simulink model "final_quadruped_040622"  (R2021a)
settings: Solver=FixedStepAuto  StartTime=0.0  StopTime=5  FixedStep=.001  RelTol=1e-3  EnableMultiTasking=on
values from neighbouring files (symbols this model uses):
  foot_x = 8    [bipedparameters.m]    (also in fcn.m; finalrobotParameters.m; finalrobotParameters_110522.m; finalrobotParameters_140522.m)
  foot_y = 6    [bipedparameters.m]    (also in fcn.m; finalrobotParameters.m; finalrobotParameters_110522.m; finalrobotParameters_140522.m)
  foot_z = 1    [bipedparameters.m]    (also in fcn.m; finalrobotParameters.m; finalrobotParameters_110522.m; finalrobotParameters_140522.m)
  height_plane = 0.025    [bipedparameters.m]    (also in finalrobotParameters.m; finalrobotParameters_110522.m; finalrobotParameters_140522.m; finalrobotParameters_240522.m)
  kd_ankle = 1000    [bipedparameters.m]    (also in finalrobotParameters_240522.m)
  kd_hip = 1000    [bipedparameters.m]    (also in finalrobotParameters_240522.m)
  kd_knee = 1000    [bipedparameters.m]    (also in finalrobotParameters_240522.m)
  ki_ankle = 1000    [bipedparameters.m]    (also in finalrobotParameters_240522.m)
  ki_hip = 1000    [bipedparameters.m]    (also in finalrobotParameters_240522.m)
  ki_knee = 2000    [bipedparameters.m]    (also in finalrobotParameters_240522.m)
  kp_ankle = 1000    [bipedparameters.m]    (also in finalrobotParameters_240522.m)
  kp_hip = 1000    [bipedparameters.m]    (also in finalrobotParameters_240522.m)
  kp_knee = 2000    [bipedparameters.m]    (also in finalrobotParameters_240522.m)
  lower_leg_length = 10    [bipedparameters.m]    (also in fcn.m; finalrobotParameters.m; finalrobotParameters_110522.m; finalrobotParameters_140522.m)
  m_ll = density*leg_radius*leg_radius*lower_leg_length*3.141592653589*0.01*0.01*0.01    (= 0.0176714586764)    [bipedparameters.m]    (also in fcn.m; finalrobotParameters_140522.m; finalrobotParameters_240522.m; hdotlb.m)
  m_ul = density*leg_radius*leg_radius*upper_leg_length*3.141592653589*0.01*0.01*0.01    (= 0.0176714586764)    [bipedparameters.m]    (also in fcn.m; finalrobotParameters_140522.m; finalrobotParameters_240522.m; hdotlb.m)
  plane_x = 25    [bipedparameters.m]    (also in finalrobotParameters.m; finalrobotParameters_110522.m; finalrobotParameters_140522.m; finalrobotParameters_240522.m)
  plane_y = 3    [bipedparameters.m]    (also in finalrobotParameters.m; finalrobotParameters_110522.m; finalrobotParameters_140522.m; finalrobotParameters_240522.m)
  torso_offset_x = -0.5    [bipedparameters.m]    (also in finalrobotParameters.m = 10; finalrobotParameters_110522.m = 10; finalrobotParameters_140522.m = 10; finalrobotParameters_240522.m = 10)
  torso_offset_z = -2    [bipedparameters.m]    (also in finalrobotParameters.m; finalrobotParameters_110522.m; finalrobotParameters_140522.m; finalrobotParameters_240522.m)
  torso_x = 5    [bipedparameters.m]    (also in fcn.m = 25; finalrobotParameters.m = 25; finalrobotParameters_110522.m = 25; finalrobotParameters_140522.m = 25)
  torso_y = 10    [bipedparameters.m]    (also in fcn.m = 16; finalrobotParameters.m = 16; finalrobotParameters_110522.m = 16; finalrobotParameters_140522.m = 16)
  torso_z = 8    [bipedparameters.m]    (also in fcn.m = 10; finalrobotParameters.m = 10; finalrobotParameters_110522.m = 10; finalrobotParameters_140522.m = 10)
  upper_leg_length = 10    [bipedparameters.m]    (also in fcn.m; finalrobotParameters.m; finalrobotParameters_110522.m; finalrobotParameters_140522.m)
undefined symbols (not defined in the file or in its folder): angleLFhip, speedLFhip, torqueLFhip, X, Y, Z
libraries: nesl_utility x151, sm_lib x71, Contact_Forces_Lib x16, pid_lib x12, fl_lib x4
(part 2 of 7)

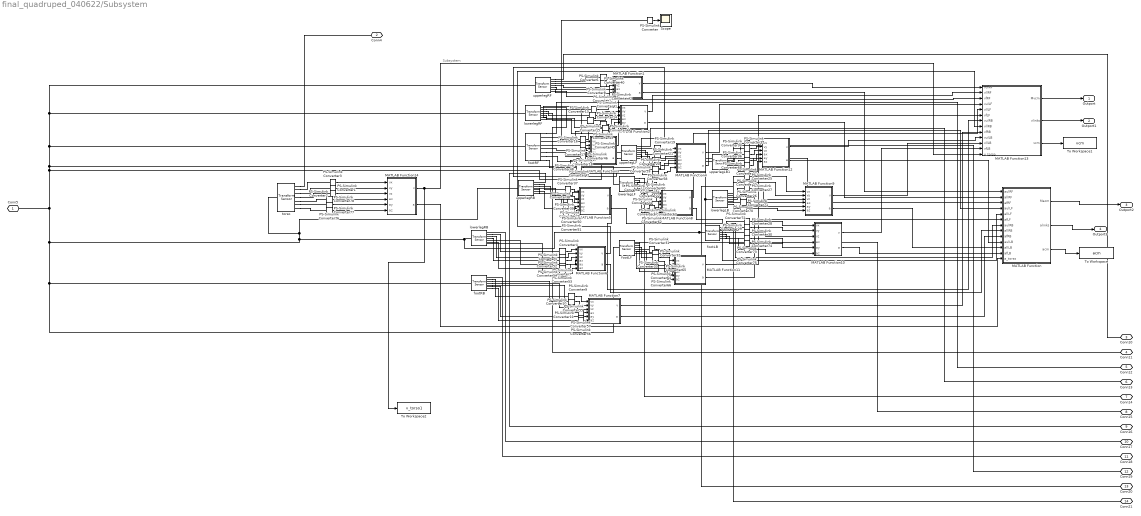
== system final_quadruped_040622/Subsystem ==
  note: Subsystem
  MATLAB Function : MATLAB Function  TreatAsAtomicUnit=on
  MATLAB Function1 : MATLAB Function  TreatAsAtomicUnit=on
  MATLAB Function10 : MATLAB Function  TreatAsAtomicUnit=on
  MATLAB Function11 : MATLAB Function  TreatAsAtomicUnit=on
  MATLAB Function12 : MATLAB Function  TreatAsAtomicUnit=on
  MATLAB Function13 : MATLAB Function  TreatAsAtomicUnit=on
  MATLAB Function14 : MATLAB Function  TreatAsAtomicUnit=on
  MATLAB Function2 : MATLAB Function  TreatAsAtomicUnit=on
  MATLAB Function3 : MATLAB Function  TreatAsAtomicUnit=on
  MATLAB Function4 : MATLAB Function  TreatAsAtomicUnit=on
  MATLAB Function5 : MATLAB Function  TreatAsAtomicUnit=on
  MATLAB Function6 : MATLAB Function  TreatAsAtomicUnit=on
  MATLAB Function7 : MATLAB Function  TreatAsAtomicUnit=on
  MATLAB Function8 : MATLAB Function  TreatAsAtomicUnit=on
  MATLAB Function9 : MATLAB Function  TreatAsAtomicUnit=on
  PS-Simulink Converter{,1..78} (79 alike) : nesl_utility/PS-Simulink Converter  PhysicalDomain=network_engine_domain  SubClassName=ps_output  LeftPortType=input  RightPortType=output  PseudoPeriodic=off  Frequencies=[]  Unit=inherit  AffineConversion=off
      settings: SourceProductBaseCode=PW,SS
  Scope : Scope
  To Workspace : ToWorkspace  VariableName=acm  SaveFormat=Timeseries  SampleTime=-1
  To Workspace1 : ToWorkspace  VariableName=vcm  SaveFormat=Timeseries  SampleTime=-1
  To Workspace2 : ToWorkspace  VariableName=v_torso1  SaveFormat=Timeseries  SampleTime=-1
  footLB : sm_lib/Frames and Transforms/Transform Sensor  MeasurementFrame=World  SenseAngle=off  SenseAxis=off  SenseAngle1=off  SenseAngle2=off  SenseAngle3=off  SenseQ=off  SenseR=off  SenseOmegaX=off  SenseOmegaY=off  SenseOmegaZ=off  SenseOmega1=off  SenseOmega2=off  SenseOmega3=off  SenseQDot=off  SenseRDot=off  SenseAlphaX=off  SenseAlphaY=off  SenseAlphaZ=off  SenseAlpha1=off  SenseAlpha2=off  SenseAlpha3=off  SenseQDDot=off  SenseRDDot=off  SenseX=off  SenseY=off  SenseZ=off  SenseRad=off  SenseAzim=off  SenseDist=off  SenseInc=off  SenseXDot=on  SenseYDot=on  SenseZDot=on  SenseRadDot=off  SenseAzimDot=off  SenseDistDot=off  SenseIncDot=off  SenseXDDot=on  SenseYDDot=on  SenseZDDot=on  SenseRadDDot=off  SenseAzimDDot=off  SenseDistDDot=off  SenseIncDDot=off
  footLF : sm_lib/Frames and Transforms/Transform Sensor  MeasurementFrame=World  SenseAngle=off  SenseAxis=off  SenseAngle1=off  SenseAngle2=off  SenseAngle3=off  SenseQ=off  SenseR=off  SenseOmegaX=off  SenseOmegaY=off  SenseOmegaZ=off  SenseOmega1=off  SenseOmega2=off  SenseOmega3=off  SenseQDot=off  SenseRDot=off  SenseAlphaX=off  SenseAlphaY=off  SenseAlphaZ=off  SenseAlpha1=off  SenseAlpha2=off  SenseAlpha3=off  SenseQDDot=off  SenseRDDot=off  SenseX=off  SenseY=off  SenseZ=off  SenseRad=off  SenseAzim=off  SenseDist=off  SenseInc=off  SenseXDot=on  SenseYDot=on  SenseZDot=on  SenseRadDot=off  SenseAzimDot=off  SenseDistDot=off  SenseIncDot=off  SenseXDDot=on  SenseYDDot=on  SenseZDDot=on  SenseRadDDot=off  SenseAzimDDot=off  SenseDistDDot=off  SenseIncDDot=off
  footRB : sm_lib/Frames and Transforms/Transform Sensor  MeasurementFrame=World  SenseAngle=off  SenseAxis=off  SenseAngle1=off  SenseAngle2=off  SenseAngle3=off  SenseQ=off  SenseR=off  SenseOmegaX=off  SenseOmegaY=off  SenseOmegaZ=off  SenseOmega1=off  SenseOmega2=off  SenseOmega3=off  SenseQDot=off  SenseRDot=off  SenseAlphaX=off  SenseAlphaY=off  SenseAlphaZ=off  SenseAlpha1=off  SenseAlpha2=off  SenseAlpha3=off  SenseQDDot=off  SenseRDDot=off  SenseX=off  SenseY=off  SenseZ=off  SenseRad=off  SenseAzim=off  SenseDist=off  SenseInc=off  SenseXDot=on  SenseYDot=on  SenseZDot=on  SenseRadDot=off  SenseAzimDot=off  SenseDistDot=off  SenseIncDot=off  SenseXDDot=on  SenseYDDot=on  SenseZDDot=on  SenseRadDDot=off  SenseAzimDDot=off  SenseDistDDot=off  SenseIncDDot=off
  footRF : sm_lib/Frames and Transforms/Transform Sensor  MeasurementFrame=World  SenseAngle=on  SenseAxis=off  SenseAngle1=off  SenseAngle2=off  SenseAngle3=off  SenseQ=off  SenseR=off  SenseOmegaX=off  SenseOmegaY=off  SenseOmegaZ=off  SenseOmega1=off  SenseOmega2=off  SenseOmega3=off  SenseQDot=off  SenseRDot=off  SenseAlphaX=off  SenseAlphaY=off  SenseAlphaZ=off  SenseAlpha1=off  SenseAlpha2=off  SenseAlpha3=off  SenseQDDot=off  SenseRDDot=off  SenseX=off  SenseY=off  SenseZ=off  SenseRad=off  SenseAzim=off  SenseDist=off  SenseInc=off  SenseXDot=on  SenseYDot=on  SenseZDot=on  SenseRadDot=off  SenseAzimDot=off  SenseDistDot=off  SenseIncDot=off  SenseXDDot=on  SenseYDDot=on  SenseZDDot=on  SenseRadDDot=off  SenseAzimDDot=off  SenseDistDDot=off  SenseIncDDot=off
  lowerlegLB : sm_lib/Frames and Transforms/Transform Sensor  MeasurementFrame=World  SenseAngle=off  SenseAxis=off  SenseAngle1=off  SenseAngle2=off  SenseAngle3=off  SenseQ=off  SenseR=off  SenseOmegaX=off  SenseOmegaY=off  SenseOmegaZ=off  SenseOmega1=off  SenseOmega2=off  SenseOmega3=off  SenseQDot=off  SenseRDot=off  SenseAlphaX=off  SenseAlphaY=off  SenseAlphaZ=off  SenseAlpha1=off  SenseAlpha2=off  SenseAlpha3=off  SenseQDDot=off  SenseRDDot=off  SenseX=off  SenseY=off  SenseZ=off  SenseRad=off  SenseAzim=off  SenseDist=off  SenseInc=off  SenseXDot=on  SenseYDot=on  SenseZDot=on  SenseRadDot=off  SenseAzimDot=off  SenseDistDot=off  SenseIncDot=off  SenseXDDot=on  SenseYDDot=on  SenseZDDot=on  SenseRadDDot=off  SenseAzimDDot=off  SenseDistDDot=off  SenseIncDDot=off
  lowerlegLF : sm_lib/Frames and Transforms/Transform Sensor  MeasurementFrame=World  SenseAngle=off  SenseAxis=off  SenseAngle1=off  SenseAngle2=off  SenseAngle3=off  SenseQ=off  SenseR=off  SenseOmegaX=off  SenseOmegaY=off  SenseOmegaZ=off  SenseOmega1=off  SenseOmega2=off  SenseOmega3=off  SenseQDot=off  SenseRDot=off  SenseAlphaX=off  SenseAlphaY=off  SenseAlphaZ=off  SenseAlpha1=off  SenseAlpha2=off  SenseAlpha3=off  SenseQDDot=off  SenseRDDot=off  SenseX=off  SenseY=off  SenseZ=off  SenseRad=off  SenseAzim=off  SenseDist=off  SenseInc=off  SenseXDot=on  SenseYDot=on  SenseZDot=on  SenseRadDot=off  SenseAzimDot=off  SenseDistDot=off  SenseIncDot=off  SenseXDDot=on  SenseYDDot=on  SenseZDDot=on  SenseRadDDot=off  SenseAzimDDot=off  SenseDistDDot=off  SenseIncDDot=off
  lowerlegRB : sm_lib/Frames and Transforms/Transform Sensor  MeasurementFrame=World  SenseAngle=off  SenseAxis=off  SenseAngle1=off  SenseAngle2=off  SenseAngle3=off  SenseQ=off  SenseR=off  SenseOmegaX=off  SenseOmegaY=off  SenseOmegaZ=off  SenseOmega1=off  SenseOmega2=off  SenseOmega3=off  SenseQDot=off  SenseRDot=off  SenseAlphaX=off  SenseAlphaY=off  SenseAlphaZ=off  SenseAlpha1=off  SenseAlpha2=off  SenseAlpha3=off  SenseQDDot=off  SenseRDDot=off  SenseX=off  SenseY=off  SenseZ=off  SenseRad=off  SenseAzim=off  SenseDist=off  SenseInc=off  SenseXDot=on  SenseYDot=on  SenseZDot=on  SenseRadDot=off  SenseAzimDot=off  SenseDistDot=off  SenseIncDot=off  SenseXDDot=on  SenseYDDot=on  SenseZDDot=on  SenseRadDDot=off  SenseAzimDDot=off  SenseDistDDot=off  SenseIncDDot=off
  lowerlegRF : sm_lib/Frames and Transforms/Transform Sensor  MeasurementFrame=World  SenseAngle=off  SenseAxis=off  SenseAngle1=off  SenseAngle2=off  SenseAngle3=off  SenseQ=off  SenseR=off  SenseOmegaX=off  SenseOmegaY=off  SenseOmegaZ=off  SenseOmega1=off  SenseOmega2=off  SenseOmega3=off  SenseQDot=off  SenseRDot=off  SenseAlphaX=off  SenseAlphaY=off  SenseAlphaZ=off  SenseAlpha1=off  SenseAlpha2=off  SenseAlpha3=off  SenseQDDot=off  SenseRDDot=off  SenseX=off  SenseY=off  SenseZ=off  SenseRad=off  SenseAzim=off  SenseDist=off  SenseInc=off  SenseXDot=on  SenseYDot=on  SenseZDot=on  SenseRadDot=off  SenseAzimDot=off  SenseDistDot=off  SenseIncDot=off  SenseXDDot=on  SenseYDDot=on  SenseZDDot=on  SenseRadDDot=off  SenseAzimDDot=off  SenseDistDDot=off  SenseIncDDot=off
  torso : sm_lib/Frames and Transforms/Transform Sensor  MeasurementFrame=World  SenseAngle=off  SenseAxis=off  SenseAngle1=off  SenseAngle2=off  SenseAngle3=off  SenseQ=off  SenseR=off  SenseOmegaX=off  SenseOmegaY=off  SenseOmegaZ=off  SenseOmega1=off  SenseOmega2=off  SenseOmega3=off  SenseQDot=off  SenseRDot=off  SenseAlphaX=off  SenseAlphaY=off  SenseAlphaZ=off  SenseAlpha1=off  SenseAlpha2=off  SenseAlpha3=off  SenseQDDot=off  SenseRDDot=off  SenseX=off  SenseY=off  SenseZ=off  SenseRad=off  SenseAzim=off  SenseDist=off  SenseInc=off  SenseXDot=on  SenseYDot=on  SenseZDot=on  SenseRadDot=off  SenseAzimDot=off  SenseDistDot=off  SenseIncDot=off  SenseXDDot=on  SenseYDDot=on  SenseZDDot=on  SenseRadDDot=off  SenseAzimDDot=off  SenseDistDDot=off  SenseIncDDot=off
  upperlegLB1 : sm_lib/Frames and Transforms/Transform Sensor  MeasurementFrame=World  SenseAngle=off  SenseAxis=off  SenseAngle1=off  SenseAngle2=off  SenseAngle3=off  SenseQ=off  SenseR=off  SenseOmegaX=off  SenseOmegaY=off  SenseOmegaZ=off  SenseOmega1=off  SenseOmega2=off  SenseOmega3=off  SenseQDot=off  SenseRDot=off  SenseAlphaX=off  SenseAlphaY=off  SenseAlphaZ=off  SenseAlpha1=off  SenseAlpha2=off  SenseAlpha3=off  SenseQDDot=off  SenseRDDot=off  SenseX=off  SenseY=off  SenseZ=off  SenseRad=off  SenseAzim=off  SenseDist=off  SenseInc=off  SenseXDot=on  SenseYDot=on  SenseZDot=on  SenseRadDot=off  SenseAzimDot=off  SenseDistDot=off  SenseIncDot=off  SenseXDDot=on  SenseYDDot=on  SenseZDDot=on  SenseRadDDot=off  SenseAzimDDot=off  SenseDistDDot=off  SenseIncDDot=off
  upperlegLF : sm_lib/Frames and Transforms/Transform Sensor  MeasurementFrame=World  SenseAngle=off  SenseAxis=off  SenseAngle1=off  SenseAngle2=off  SenseAngle3=off  SenseQ=off  SenseR=off  SenseOmegaX=off  SenseOmegaY=off  SenseOmegaZ=off  SenseOmega1=off  SenseOmega2=off  SenseOmega3=off  SenseQDot=off  SenseRDot=off  SenseAlphaX=off  SenseAlphaY=off  SenseAlphaZ=off  SenseAlpha1=off  SenseAlpha2=off  SenseAlpha3=off  SenseQDDot=off  SenseRDDot=off  SenseX=off  SenseY=off  SenseZ=off  SenseRad=off  SenseAzim=off  SenseDist=off  SenseInc=off  SenseXDot=on  SenseYDot=on  SenseZDot=on  SenseRadDot=off  SenseAzimDot=off  SenseDistDot=off  SenseIncDot=off  SenseXDDot=on  SenseYDDot=on  SenseZDDot=on  SenseRadDDot=off  SenseAzimDDot=off  SenseDistDDot=off  SenseIncDDot=off
  upperlegRB : sm_lib/Frames and Transforms/Transform Sensor  MeasurementFrame=World  SenseAngle=off  SenseAxis=off  SenseAngle1=off  SenseAngle2=off  SenseAngle3=off  SenseQ=off  SenseR=off  SenseOmegaX=off  SenseOmegaY=off  SenseOmegaZ=off  SenseOmega1=off  SenseOmega2=off  SenseOmega3=off  SenseQDot=off  SenseRDot=off  SenseAlphaX=off  SenseAlphaY=off  SenseAlphaZ=off  SenseAlpha1=off  SenseAlpha2=off  SenseAlpha3=off  SenseQDDot=off  SenseRDDot=off  SenseX=off  SenseY=off  SenseZ=off  SenseRad=off  SenseAzim=off  SenseDist=off  SenseInc=off  SenseXDot=on  SenseYDot=on  SenseZDot=on  SenseRadDot=off  SenseAzimDot=off  SenseDistDot=off  SenseIncDot=off  SenseXDDot=on  SenseYDDot=on  SenseZDDot=on  SenseRadDDot=off  SenseAzimDDot=off  SenseDistDDot=off  SenseIncDDot=off
  upperlegRF : sm_lib/Frames and Transforms/Transform Sensor  MeasurementFrame=World  SenseAngle=off  SenseAxis=off  SenseAngle1=off  SenseAngle2=off  SenseAngle3=off  SenseQ=off  SenseR=off  SenseOmegaX=off  SenseOmegaY=off  SenseOmegaZ=off  SenseOmega1=off  SenseOmega2=off  SenseOmega3=off  SenseQDot=off  SenseRDot=off  SenseAlphaX=off  SenseAlphaY=off  SenseAlphaZ=off  SenseAlpha1=off  SenseAlpha2=off  SenseAlpha3=off  SenseQDDot=off  SenseRDDot=off  SenseX=off  SenseY=off  SenseZ=off  SenseRad=off  SenseAzim=off  SenseDist=off  SenseInc=off  SenseXDot=on  SenseYDot=on  SenseZDot=on  SenseRadDot=off  SenseAzimDot=off  SenseDistDot=off  SenseIncDot=off  SenseXDDot=on  SenseYDDot=on  SenseZDDot=on  SenseRadDDot=off  SenseAzimDDot=off  SenseDistDDot=off  SenseIncDDot=off
  Conn5 : PMIOPort  Side=Left
  Conn4 : PMIOPort  Port=2  Side=Right
  Conn10 : PMIOPort  Port=3  Side=Right
  Conn11 : PMIOPort  Port=4  Side=Right
  Conn12 : PMIOPort  Port=5  Side=Right
  Conn13 : PMIOPort  Port=6  Side=Right
  Conn14 : PMIOPort  Port=7  Side=Right
  Conn15 : PMIOPort  Port=8  Side=Right
  Conn16 : PMIOPort  Port=9  Side=Right
  Conn17 : PMIOPort  Port=10  Side=Right
  Conn18 : PMIOPort  Port=11  Side=Right
  Conn19 : PMIOPort  Port=12  Side=Right
  Conn20 : PMIOPort  Port=13  Side=Right
  Conn21 : PMIOPort  Port=14  Side=Right
  Outport : Outport
  Outport1 : Outport  Port=2
  Outport2 : Outport  Port=3
  Outport3 : Outport  Port=4
  wires:
  PS-Simulink Converter10/1 -> MATLAB Function7/2(vy)
  PS-Simulink Converter13/1 -> MATLAB Function2/1(vx)
  MATLAB Function12/1(v) -> MATLAB Function13/10(vulLB)
  PS-Simulink Converter36/1 -> MATLAB Function12/3(vz)
  PS-Simulink Converter14/1 -> MATLAB Function2/2(vy)
  PS-Simulink Converter9/1 -> MATLAB Function7/1(vx)
  PS-Simulink Converter11/1 -> MATLAB Function7/3(vz)
  PS-Simulink Converter8/1 -> MATLAB Function1/2(vy)
  PS-Simulink Converter7/1 -> MATLAB Function6/3(vz)
  PS-Simulink Converter38/1 -> MATLAB Function5/2(vy)
  PS-Simulink Converter16/1 -> MATLAB Function3/1(vx)
  MATLAB Function9/1(v) -> MATLAB Function13/11(vllLB)
  MATLAB Function1/1(v) -> MATLAB Function13/1(vulRF)
  PS-Simulink Converter17/1 -> MATLAB Function3/2(vy)
  PS-Simulink Converter28/1 -> MATLAB Function10/1(vx)
  PS-Simulink Converter21/1 -> MATLAB Function4/3(vz)
  PS-Simulink Converter18/1 -> MATLAB Function3/3(vz)
  PS-Simulink Converter6/1 -> MATLAB Function1/1(vx)
  PS-Simulink Converter19/1 -> MATLAB Function4/1(vx)
  PS-Simulink Converter5/1 -> MATLAB Function6/2(vy)
  PS-Simulink Converter20/1 -> MATLAB Function4/2(vy)
  PS-Simulink Converter12/1 -> MATLAB Function1/3(vz)
  PS-Simulink Converter15/1 -> MATLAB Function2/3(vz)
  PS-Simulink Converter39/1 -> MATLAB Function5/3(vz)
  MATLAB Function2/1(v) -> MATLAB Function13/2(vllRF)
  MATLAB Function10/1(v) -> MATLAB Function13/12(vfLB)
  PS-Simulink Converter27/1 -> MATLAB Function9/3(vz)
  PS-Simulink Converter4/1 -> MATLAB Function6/1(vx)
  PS-Simulink Converter25/1 -> MATLAB Function9/1(vx)
  PS-Simulink Converter37/1 -> MATLAB Function5/1(vx)
  PS-Simulink Converter26/1 -> MATLAB Function9/2(vy)
  PS-Simulink Converter24/1 -> MATLAB Function8/3(vz)
  PS-Simulink Converter22/1 -> MATLAB Function8/1(vx)
  PS-Simulink Converter23/1 -> MATLAB Function8/2(vy)
  PS-Simulink Converter34/1 -> MATLAB Function12/1(vx)
  PS-Simulink Converter35/1 -> MATLAB Function12/2(vy)
  MATLAB Function7/1(v) -> MATLAB Function13/9(vfRB)
  MATLAB Function6/1(v) -> MATLAB Function13/8(vllRB)
  MATLAB Function5/1(v) -> MATLAB Function13/7(vulRB)
  MATLAB Function11/1(v) -> MATLAB Function13/6(vfLF)
  PS-Simulink Converter33/1 -> MATLAB Function11/3(vz)
  MATLAB Function8/1(v) -> MATLAB Function13/5(vllLF)
  MATLAB Function4/1(v) -> MATLAB Function13/4(vulLF)
  MATLAB Function3/1(v) -> MATLAB Function13/3(vfRF)
  PS-Simulink Converter32/1 -> MATLAB Function11/2(vy)
  PS-Simulink Converter31/1 -> MATLAB Function11/1(vx)
  PS-Simulink Converter30/1 -> MATLAB Function10/3(vz)
  PS-Simulink Converter29/1 -> MATLAB Function10/2(vy)
  PS-Simulink Converter3/1 -> MATLAB Function14/1(vx)
  PS-Simulink Converter1/1 -> MATLAB Function14/2(vy)
  PS-Simulink Converter2/1 -> MATLAB Function14/3(vz)
  MATLAB Function14/1(v) -> To Workspace2/1, MATLAB Function13/13(v_torso)
  MATLAB Function13/1(Mvcm) -> Outport/1
  MATLAB Function13/2(vlinks) -> Outport1/1
  PS-Simulink Converter/1 -> Scope/1
  PS-Simulink Converter40/1 -> MATLAB Function1/4(ax)
  PS-Simulink Converter41/1 -> MATLAB Function1/5(ay)
  PS-Simulink Converter42/1 -> MATLAB Function1/6(az)
  PS-Simulink Converter43/1 -> MATLAB Function2/4(ax)
  PS-Simulink Converter44/1 -> MATLAB Function2/5(ay)
  PS-Simulink Converter45/1 -> MATLAB Function2/6(az)
  PS-Simulink Converter46/1 -> MATLAB Function3/4(ax)
  PS-Simulink Converter47/1 -> MATLAB Function3/5(ay)
  PS-Simulink Converter48/1 -> MATLAB Function3/6(az)
  PS-Simulink Converter49/1 -> MATLAB Function5/4(ax)
  PS-Simulink Converter50/1 -> MATLAB Function5/5(ay)
  PS-Simulink Converter51/1 -> MATLAB Function5/6(az)
  PS-Simulink Converter52/1 -> MATLAB Function6/4(ax)
  PS-Simulink Converter53/1 -> MATLAB Function6/5(ay)
  PS-Simulink Converter54/1 -> MATLAB Function6/6(az)
  PS-Simulink Converter55/1 -> MATLAB Function7/5(ay)
  PS-Simulink Converter57/1 -> MATLAB Function7/4(ax)
  PS-Simulink Converter56/1 -> MATLAB Function7/6(az)
  PS-Simulink Converter58/1 -> MATLAB Function4/4(ax)
  PS-Simulink Converter59/1 -> MATLAB Function4/5(ay)
  PS-Simulink Converter60/1 -> MATLAB Function4/6(az)
  PS-Simulink Converter61/1 -> MATLAB Function8/4(ax)
  PS-Simulink Converter62/1 -> MATLAB Function8/5(ay)
  PS-Simulink Converter63/1 -> MATLAB Function8/6(az)
  PS-Simulink Converter64/1 -> MATLAB Function11/4(ax)
  PS-Simulink Converter65/1 -> MATLAB Function11/5(ay)
  PS-Simulink Converter66/1 -> MATLAB Function11/6(az)
  PS-Simulink Converter67/1 -> MATLAB Function12/4(ax)
  PS-Simulink Converter68/1 -> MATLAB Function12/5(ay)
  PS-Simulink Converter69/1 -> MATLAB Function12/6(az)
  PS-Simulink Converter70/1 -> MATLAB Function9/4(ax)
  PS-Simulink Converter71/1 -> MATLAB Function9/5(ay)
  PS-Simulink Converter72/1 -> MATLAB Function9/6(az)
  PS-Simulink Converter73/1 -> MATLAB Function10/4(ax)
  PS-Simulink Converter74/1 -> MATLAB Function10/5(ay)
  PS-Simulink Converter75/1 -> MATLAB Function10/6(az)
  PS-Simulink Converter78/1 -> MATLAB Function14/4(ax)
  PS-Simulink Converter76/1 -> MATLAB Function14/5(ay)
  PS-Simulink Converter77/1 -> MATLAB Function14/6(az)
  MATLAB Function14/2(a) -> MATLAB Function/13(a_torso)
  MATLAB Function1/2(a) -> MATLAB Function/1(aulRF)
  MATLAB Function2/2(a) -> MATLAB Function/2(allRF)
  MATLAB Function3/2(a) -> MATLAB Function/3(afRF)
  MATLAB Function4/2(a) -> MATLAB Function/4(aulLF)
  MATLAB Function8/2(a) -> MATLAB Function/5(allLF)
  MATLAB Function11/2(a) -> MATLAB Function/6(afLF)
  MATLAB Function5/2(a) -> MATLAB Function/7(aulRB)
  MATLAB Function6/2(a) -> MATLAB Function/8(allRB)
  MATLAB Function7/2(a) -> MATLAB Function/9(afRB)
  MATLAB Function12/2(a) -> MATLAB Function/10(aulLB)
  MATLAB Function9/2(a) -> MATLAB Function/11(allLB)
  MATLAB Function10/2(a) -> MATLAB Function/12(afLB)
  MATLAB Function/1(Macm) -> Outport2/1
  MATLAB Function/2(alinks) -> Outport3/1
  MATLAB Function/3(acm) -> To Workspace/1
  MATLAB Function13/3(vcm) -> To Workspace1/1
  connections:
  footRB/RConn4 -- PS-Simulink Converter11/LConn1
  lowerlegLF/RConn2 -- PS-Simulink Converter22/LConn1
  upperlegLF/RConn4 -- PS-Simulink Converter21/LConn1
  footLB/RConn2 -- PS-Simulink Converter28/LConn1
  upperlegLB1/RConn1 -- Conn19/RConn1
  footLF/RConn2 -- PS-Simulink Converter31/LConn1
  lowerlegLB/LConn1 -- upperlegLB1/LConn1 -- footLB/LConn1 -- torso/LConn1 -- upperlegRB/LConn1 -- footLF/LConn1 -- footRB/LConn1 -- upperlegRF/LConn1 -- lowerlegRF/LConn1 -- footRF/LConn1 -- lowerlegLF/LConn1 -- upperlegLF/LConn1 -- Conn5/RConn1 -- lowerlegRB/LConn1
  lowerlegRB/RConn4 -- PS-Simulink Converter7/LConn1
  Conn17/RConn1 -- lowerlegRB/RConn1
  upperlegLF/RConn2 -- PS-Simulink Converter19/LConn1
  upperlegLF/RConn3 -- PS-Simulink Converter20/LConn1
  lowerlegRF/RConn3 -- PS-Simulink Converter14/LConn1
  footLB/RConn4 -- PS-Simulink Converter30/LConn1
  footRB/RConn3 -- PS-Simulink Converter10/LConn1
  upperlegRB/RConn3 -- PS-Simulink Converter38/LConn1
  lowerlegRF/RConn2 -- PS-Simulink Converter13/LConn1
  upperlegRB/RConn4 -- PS-Simulink Converter39/LConn1
  upperlegRB/RConn2 -- PS-Simulink Converter37/LConn1
  upperlegRF/RConn2 -- PS-Simulink Converter6/LConn1
  footLB/RConn1 -- Conn21/RConn1
  lowerlegRF/RConn4 -- PS-Simulink Converter15/LConn1
  lowerlegLF/RConn4 -- PS-Simulink Converter24/LConn1
  upperlegLB1/RConn4 -- PS-Simulink Converter36/LConn1
  footRB/RConn2 -- PS-Simulink Converter9/LConn1
  upperlegRF/RConn4 -- PS-Simulink Converter12/LConn1
  upperlegRF/RConn3 -- PS-Simulink Converter8/LConn1
  lowerlegLF/RConn3 -- PS-Simulink Converter23/LConn1
  lowerlegRB/RConn3 -- PS-Simulink Converter5/LConn1
  lowerlegRB/RConn2 -- PS-Simulink Converter4/LConn1
  lowerlegLB/RConn3 -- PS-Simulink Converter26/LConn1
  lowerlegLB/RConn4 -- PS-Simulink Converter27/LConn1
  lowerlegLB/RConn2 -- PS-Simulink Converter25/LConn1
  lowerlegLB/RConn1 -- Conn20/RConn1
  upperlegLB1/RConn3 -- PS-Simulink Converter35/LConn1
  upperlegLB1/RConn2 -- PS-Simulink Converter34/LConn1
  upperlegRF/RConn1 -- Conn10/RConn1
  upperlegLF/RConn1 -- Conn13/RConn1
  footLF/RConn3 -- PS-Simulink Converter32/LConn1
  footLF/RConn4 -- PS-Simulink Converter33/LConn1
  footLB/RConn3 -- PS-Simulink Converter29/LConn1
  Conn18/RConn1 -- footRB/RConn1
  footLF/RConn1 -- Conn15/RConn1
  Conn16/RConn1 -- upperlegRB/RConn1
  lowerlegLF/RConn1 -- Conn14/RConn1
  Conn11/RConn1 -- lowerlegRF/RConn1
  footRF/RConn1 -- Conn12/RConn1
  torso/RConn1 -- Conn4/RConn1
  torso/RConn3 -- PS-Simulink Converter1/LConn1
  torso/RConn2 -- PS-Simulink Converter3/LConn1
  torso/RConn4 -- PS-Simulink Converter2/LConn1
  PS-Simulink Converter16/LConn1 -- footRF/RConn3
  PS-Simulink Converter17/LConn1 -- footRF/RConn4
  PS-Simulink Converter18/LConn1 -- footRF/RConn5
  PS-Simulink Converter/LConn1 -- footRF/RConn2
  upperlegRF/RConn5 -- PS-Simulink Converter40/LConn1
  upperlegRF/RConn6 -- PS-Simulink Converter41/LConn1
  upperlegRF/RConn7 -- PS-Simulink Converter42/LConn1
  lowerlegRF/RConn5 -- PS-Simulink Converter43/LConn1
  lowerlegRF/RConn6 -- PS-Simulink Converter44/LConn1
  lowerlegRF/RConn7 -- PS-Simulink Converter45/LConn1
  footRF/RConn6 -- PS-Simulink Converter46/LConn1
  footRF/RConn7 -- PS-Simulink Converter47/LConn1
  footRF/RConn8 -- PS-Simulink Converter48/LConn1
  upperlegRB/RConn5 -- PS-Simulink Converter49/LConn1
  upperlegRB/RConn6 -- PS-Simulink Converter50/LConn1
  upperlegRB/RConn7 -- PS-Simulink Converter51/LConn1
  PS-Simulink Converter52/LConn1 -- lowerlegRB/RConn5
  PS-Simulink Converter53/LConn1 -- lowerlegRB/RConn6
  PS-Simulink Converter54/LConn1 -- lowerlegRB/RConn7
  footRB/RConn5 -- PS-Simulink Converter57/LConn1
  footRB/RConn6 -- PS-Simulink Converter55/LConn1
  footRB/RConn7 -- PS-Simulink Converter56/LConn1
  upperlegLF/RConn5 -- PS-Simulink Converter58/LConn1
  upperlegLF/RConn6 -- PS-Simulink Converter59/LConn1
  upperlegLF/RConn7 -- PS-Simulink Converter60/LConn1
  lowerlegLF/RConn5 -- PS-Simulink Converter61/LConn1
  lowerlegLF/RConn6 -- PS-Simulink Converter62/LConn1
  lowerlegLF/RConn7 -- PS-Simulink Converter63/LConn1
  footLF/RConn5 -- PS-Simulink Converter64/LConn1
  footLF/RConn6 -- PS-Simulink Converter65/LConn1
  footLF/RConn7 -- PS-Simulink Converter66/LConn1
  upperlegLB1/RConn5 -- PS-Simulink Converter67/LConn1
  upperlegLB1/RConn6 -- PS-Simulink Converter68/LConn1
  upperlegLB1/RConn7 -- PS-Simulink Converter69/LConn1
  lowerlegLB/RConn5 -- PS-Simulink Converter70/LConn1
  lowerlegLB/RConn6 -- PS-Simulink Converter71/LConn1
  lowerlegLB/RConn7 -- PS-Simulink Converter72/LConn1
  footLB/RConn5 -- PS-Simulink Converter73/LConn1
  footLB/RConn6 -- PS-Simulink Converter74/LConn1
  footLB/RConn7 -- PS-Simulink Converter75/LConn1
  torso/RConn5 -- PS-Simulink Converter78/LConn1
  torso/RConn6 -- PS-Simulink Converter76/LConn1
  torso/RConn7 -- PS-Simulink Converter77/LConn1

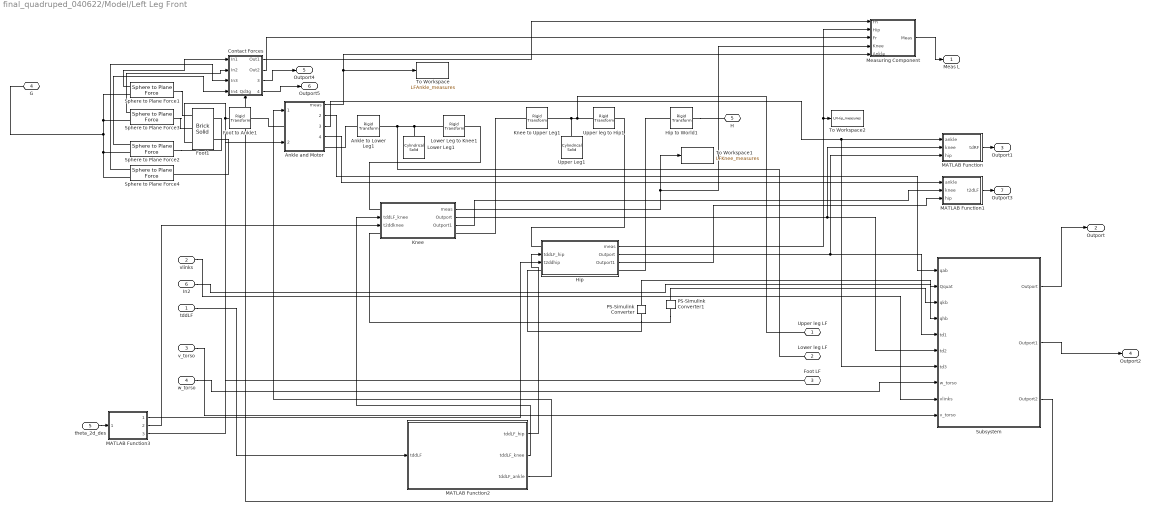
== system final_quadruped_040622/Model/Left Leg Front ==
  tddLF : Inport
  vlinks : Inport  Port=2
  v_torso : Inport  Port=3
  w_torso : Inport  Port=4
  theta_2d_des : Inport  Port=5
  In2 : Inport  Port=6
  Ankle and Motor : Subsystem
      settings: PortSchema="{\"entries\":[{\"content\":{\"sides\":[{\"content\":{\"connectorIds\":[\"In1\",\"LConn1\",\"In2\"]},\"type\":\"ConnectorPlacement.EquallySpacedRectSide\",\"uuid\":\"8820d672-3cef-4e81-999d-8ce69d7112c4\"},{\"content\":{\"connectorIds\":[\"Out1\",\"Out2\",\"Out3\",\"Out4\",\"RConn1\"],\"side\":\"RIGHT\"},\"type\":\"ConnectorPlacement.EquallySpacedRectSide\",\"uuid\":\"2ab010ff-dc37-45a7-8249-0a0b10f28039\"},{\"content\":{\"connectorIds\":[],\"side\":\"TOP\"},\"type\":\"ConnectorPlacement.EquallySpacedRectSide\",\"uuid\":\"2949f9ef-a473-4fca-9f6b-f5ba56dbec95\"}]},\"type\":\"ConnectorPlacement.EquallySpacedConnector\",\"uuid\":\"7b6aa300-a222-434d-a157-d54fa47a17c2\"}],\"packageUris\":[\"http://schema.mathworks.com/mf0/Connector/R2020b\"],\"version\":\"1.0\"}"
  Ankle to Lower Leg1 : sm_lib/Frames and Transforms/Rigid Transform  TranslationMethod=Cartesian  TranslationStandardOffset=5  TranslationLengthUnit=cm  TranslationStandardAxis=+Y  TranslationCartesianOffset=[0 lower_leg_length/2 0]  TranslationROffset=0  TranslationROffsetUnits=m  TranslationZOffset=0  TranslationZOffsetUnits=m  TranslationThetaOffset=0  TranslationThetaOffsetUnits=deg  RotationMethod=StandardAxis  RotationAngleUnits=deg  RotationStandardAxis=-X  RotationAngle=90  RotationArbitraryAxis=[0 0 1]  FollAlignAxisA=+X  BaseAlignAxisA=+Y  FollAlignAxisB=+Y  BaseAlignAxisB=+Z  RotationSequenceAxes=FollowerAxes  RotationSequence=XYX  RotationSequenceAngles=[0 0 0]  RotationSequenceAnglesUnits=deg  RotationMatrix=[1 0 0; 0 1 0; 0 0 1]
  "Contact Forces " : Subsystem
      settings: PortSchema="{\"entries\":[{\"content\":{\"sides\":[{\"content\":{\"connectorIds\":[\"In1\",\"In2\",\"In3\",\"In4\"]},\"type\":\"ConnectorPlacement.EquallySpacedRectSide\",\"uuid\":\"092bab02-781e-4e8b-aeea-5de78c3a7c59\"},{\"content\":{\"connectorIds\":[\"Out1\",\"Out2\",\"Out3\",\"Out4\"],\"side\":\"RIGHT\"},\"type\":\"ConnectorPlacement.EquallySpacedRectSide\",\"uuid\":\"1414f239-400a-4e7a-8cfa-bc0efd263a34\"},{\"content\":{\"connectorIds\":[],\"side\":\"TOP\"},\"type\":\"ConnectorPlacement.EquallySpacedRectSide\",\"uuid\":\"08c81ad5-eae1-4818-9216-87e77fef6e85\"},{\"content\":{\"connectorIds\":[\"In5\"],\"side\":\"BOTTOM\"},\"type\":\"ConnectorPlacement.EquallySpacedRectSide\",\"uuid\":\"68de5e6c-9c3a-4c3f-9e89-3545a6b6c214\"}]},\"type\":\"ConnectorPlacement.EquallySpacedConnector\",\"uuid\":\"11ab48ab-4eae-444e-84a8-984acdbad2c5\"}],\"packageUris\":[\"http://schema.mathworks.com/mf0/Connector/R2020b\"],\"version\":\"1.0\"}"
  Foot to Ankle1 : sm_lib/Frames and Transforms/Rigid Transform  TranslationMethod=Cartesian  TranslationStandardOffset=0  TranslationLengthUnit=cm  TranslationStandardAxis=+Z  TranslationCartesianOffset=foot_offset  TranslationROffset=0  TranslationROffsetUnits=m  TranslationZOffset=0  TranslationZOffsetUnits=m  TranslationThetaOffset=0  TranslationThetaOffsetUnits=deg  RotationMethod=None  RotationAngleUnits=deg  RotationStandardAxis=+X  RotationAngle=90  RotationArbitraryAxis=[0 0 1]  FollAlignAxisA=+X  BaseAlignAxisA=+Y  FollAlignAxisB=+Y  BaseAlignAxisB=+Z  RotationSequenceAxes=FollowerAxes  RotationSequence=XYX  RotationSequenceAngles=[0 0 0]  RotationSequenceAnglesUnits=deg  RotationMatrix=[1 0 0; 0 1 0; 0 0 1]
  Foot1 : sm_lib/Body Elements/Brick Solid  GraphicAmbientColor=[0.15 0.15 0.15 1.0]  BasedOnType=Density  BrickDimensions=[foot_x foot_y foot_z]  BrickDimensionUnits=cm  CenterOfMass=[0 0 0]  CenterOfMassUnits=m  GraphicDiffuseColor=[0.5 0.5 0.5]  Density=2000  DensityUnits=kg/m^3  DoExposeReferenceFrame=off  GraphicEmissiveColor=[0.0 0.0 0.0 1.0]  ExportEntireGeometry=off  SerializedFrames=<Frames><Frame><Id>Frame1</Id><Value><Name>F1</Name><Origin><Source>GeometricFeature</Source><FeatureName>+x -y -z point</FeatureName></Origin><PrimaryAxis><DefinedDirection>+Z</DefinedDirection><Source>ReferenceFrame</Source><SourceDirection>+Z</SourceDirection><FeatureName></FeatureName></PrimaryAxis><SecondaryAxis><DefinedDirection>+X</DefinedDirection><Source>ReferenceFrame</Source><SourceDirection>+X</SourceDirection><FeatureName></FeatureName></SecondaryAxis></Value></Frame><Frame><Id>Frame2</Id><Value><Name>F2</Name><Origin><Source>GeometricFeature</Source><FeatureName>+x +y -z point</FeatureName></Origin><PrimaryAxis><DefinedDirection>+Z</DefinedDirection><Source>ReferenceFrame</Source><SourceDirection>+Z</SourceDirection><FeatureName></FeatureName></PrimaryAxis><SecondaryAxis><DefinedDirection>+X</DefinedDirection><Source>ReferenceFrame</Source><SourceDirection>+X</SourceDirection><FeatureName></FeatureName></SecondaryAxis></Value></Frame><Frame><Id>Frame3</Id><Value><Name>F3</Name><Origin><Source>GeometricFeature</Source><FeatureName>-x -y -z point</FeatureName></Origin><PrimaryAxis><DefinedDirection>+Z</DefinedDirection><Source>ReferenceFrame</Source><SourceDirection>+Z</SourceDirection><FeatureName></FeatureName></PrimaryAxis><SecondaryAxis><DefinedDirection>+X</DefinedDirection><Source>ReferenceFrame</Source><SourceDirection>+X</SourceDirection><FeatureName></FeatureName></SecondaryAxis></Value></Frame><Frame><Id>Frame4</Id><Value><Name>F4</Name><Origin><Source>GeometricFeature</Source><FeatureName>-x +y -z point</FeatureName></Origin><PrimaryAxis><DefinedDirection>+Z</DefinedDirection><Source>ReferenceFrame</Source><SourceDirection>+Z</SourceDirection><FeatureName></FeatureName></PrimaryAxis><SecondaryAxis><DefinedDirection>+X</DefinedDirection><Source>ReferenceFrame</Source><SourceDirection>+X</SourceDirection><FeatureName></FeatureName></SecondaryAxis></Value></Frame><Frame><Id>Frame5</Id><Value><Name>B</Name><Origin><Source>GeometricFeature</Source><FeatureName>+z surface</FeatureName></Origin><PrimaryAxis><DefinedDirection>+Z</DefinedDirection><Source>ReferenceFrame</Source><SourceDirection>-Y</SourceDirection><FeatureName></FeatureName></PrimaryAxis><SecondaryAxis><DefinedDirection>+X</DefinedDirection><Source>ReferenceFrame</Source><SourceDirection>+X</SourceDirection><FeatureName></FeatureName></SecondaryAxis></Value></Frame></Frames>  MarkerShape=Sphere  MarkerSize=10  GraphicType=FromGeometry  InertiaType=CalculateFromGeometry  Mass=1  MassUnits=kg  MomentsOfInertia=[1 1 1]  MomentsOfInertiaUnits=kg*m^2  GraphicOpacity=1.0  ProductsOfInertia=[1 1 1]  ProductsOfInertiaUnits=kg*m^2  GraphicShininess=75  GraphicSpecularColor=[0.5 0.5 0.5 1.0]  GraphicVisPropType=SimpleVisualProperties
  Hip : Subsystem
      settings: PortSchema="{\"entries\":[{\"content\":{\"sides\":[{\"content\":{\"connectorIds\":[\"LConn1\",\"In1\",\"In2\",\"LConn2\"]},\"type\":\"ConnectorPlacement.EquallySpacedRectSide\",\"uuid\":\"3c672348-e331-4589-83a8-aa84cb04ec22\"},{\"content\":{\"connectorIds\":[\"Out1\",\"Out2\",\"Out3\",\"RConn1\"],\"side\":\"RIGHT\"},\"type\":\"ConnectorPlacement.EquallySpacedRectSide\",\"uuid\":\"0cc20eac-f861-4ef7-921b-23889a7eea47\"},{\"content\":{\"connectorIds\":[],\"side\":\"TOP\"},\"type\":\"ConnectorPlacement.EquallySpacedRectSide\",\"uuid\":\"90940c46-a35e-4cbd-8c5c-08301adb8b47\"}]},\"type\":\"ConnectorPlacement.EquallySpacedConnector\",\"uuid\":\"ac1266b5-f3f5-41bb-99c9-3c0745f7848a\"}],\"packageUris\":[\"http://schema.mathworks.com/mf0/Connector/R2020b\"],\"version\":\"1.0\"}"
  Hip to World1 : sm_lib/Frames and Transforms/Rigid Transform  TranslationMethod=None  TranslationStandardOffset=0  TranslationLengthUnit=m  TranslationStandardAxis=+Z  TranslationCartesianOffset=[0 0 0]  TranslationROffset=0  TranslationROffsetUnits=m  TranslationZOffset=0  TranslationZOffsetUnits=m  TranslationThetaOffset=0  TranslationThetaOffsetUnits=deg  RotationMethod=StandardAxis  RotationAngleUnits=deg  RotationStandardAxis=+X  RotationAngle=-90  RotationArbitraryAxis=[0 0 1]  FollAlignAxisA=+X  BaseAlignAxisA=+Y  FollAlignAxisB=+Y  BaseAlignAxisB=+Z  RotationSequenceAxes=FollowerAxes  RotationSequence=XYX  RotationSequenceAngles=[0 0 0]  RotationSequenceAnglesUnits=deg  RotationMatrix=[1 0 0; 0 1 0; 0 0 1]
  Knee : Subsystem
      settings: PortSchema="{\"entries\":[{\"content\":{\"sides\":[{\"content\":{\"connectorIds\":[\"LConn1\",\"In1\",\"In2\",\"LConn2\"]},\"type\":\"ConnectorPlacement.EquallySpacedRectSide\",\"uuid\":\"3c672348-e331-4589-83a8-aa84cb04ec22\"},{\"content\":{\"connectorIds\":[\"Out1\",\"Out2\",\"Out3\",\"RConn1\"],\"side\":\"RIGHT\"},\"type\":\"ConnectorPlacement.EquallySpacedRectSide\",\"uuid\":\"0cc20eac-f861-4ef7-921b-23889a7eea47\"},{\"content\":{\"connectorIds\":[],\"side\":\"TOP\"},\"type\":\"ConnectorPlacement.EquallySpacedRectSide\",\"uuid\":\"90940c46-a35e-4cbd-8c5c-08301adb8b47\"}]},\"type\":\"ConnectorPlacement.EquallySpacedConnector\",\"uuid\":\"ac1266b5-f3f5-41bb-99c9-3c0745f7848a\"}],\"packageUris\":[\"http://schema.mathworks.com/mf0/Connector/R2020b\"],\"version\":\"1.0\"}"
  Knee to Upper Leg1 : sm_lib/Frames and Transforms/Rigid Transform  TranslationMethod=Cartesian  TranslationStandardOffset=5  TranslationLengthUnit=cm  TranslationStandardAxis=+Y  TranslationCartesianOffset=[0 upper_leg_length/2 0]  TranslationROffset=0  TranslationROffsetUnits=m  TranslationZOffset=0  TranslationZOffsetUnits=m  TranslationThetaOffset=0  TranslationThetaOffsetUnits=deg  RotationMethod=StandardAxis  RotationAngleUnits=deg  RotationStandardAxis=+X  RotationAngle=-90  RotationArbitraryAxis=[0 0 1]  FollAlignAxisA=+X  BaseAlignAxisA=+Y  FollAlignAxisB=+Y  BaseAlignAxisB=+Z  RotationSequenceAxes=FollowerAxes  RotationSequence=XYX  RotationSequenceAngles=[0 0 0]  RotationSequenceAnglesUnits=deg  RotationMatrix=[1 0 0; 0 1 0; 0 0 1]
  Lower Leg1 : sm_lib/Body Elements/Cylindrical Solid  GraphicAmbientColor=[0.15 0.15 0.15 1.0]  BasedOnType=Density  CenterOfMass=[0 0 0]  CenterOfMassUnits=m  GraphicDiffuseColor=[0.5 0.5 0.5]  CylinderLength=lower_leg_length  CylinderLengthUnits=cm  CylinderRadius=leg_radius  CylinderRadiusUnits=cm  Density=1000  DensityUnits=kg/m^3  DoExposeReferenceFrame=on  GraphicEmissiveColor=[0.0 0.0 0.0 1.0]  ExportEntireGeometry=off  SerializedFrames=<Frames/>  MarkerShape=Sphere  MarkerSize=10  GraphicType=FromGeometry  InertiaType=CalculateFromGeometry  Mass=1  MassUnits=kg  MomentsOfInertia=[1 1 1]  MomentsOfInertiaUnits=kg*m^2  GraphicOpacity=1.0  ProductsOfInertia=[1 1 1]  ProductsOfInertiaUnits=kg*m^2  GraphicShininess=75  GraphicSpecularColor=[0.5 0.5 0.5 1.0]  GraphicVisPropType=SimpleVisualProperties
  Lower Leg to Knee1 : sm_lib/Frames and Transforms/Rigid Transform  TranslationMethod=Cartesian  TranslationStandardOffset=5  TranslationLengthUnit=cm  TranslationStandardAxis=+Z  TranslationCartesianOffset=[0 0 lower_leg_length/2]  TranslationROffset=0  TranslationROffsetUnits=m  TranslationZOffset=0  TranslationZOffsetUnits=m  TranslationThetaOffset=0  TranslationThetaOffsetUnits=deg  RotationMethod=StandardAxis  RotationAngleUnits=deg  RotationStandardAxis=+X  RotationAngle=90  RotationArbitraryAxis=[0 0 1]  FollAlignAxisA=+X  BaseAlignAxisA=+Y  FollAlignAxisB=+Y  BaseAlignAxisB=+Z  RotationSequenceAxes=FollowerAxes  RotationSequence=XYX  RotationSequenceAngles=[0 0 0]  RotationSequenceAnglesUnits=deg  RotationMatrix=[1 0 0; 0 1 0; 0 0 1]
  MATLAB Function : MATLAB Function  TreatAsAtomicUnit=on
  MATLAB Function1 : MATLAB Function  TreatAsAtomicUnit=on
  MATLAB Function2 : MATLAB Function  TreatAsAtomicUnit=on
  MATLAB Function3 : MATLAB Function  TreatAsAtomicUnit=on
  Measuring Component : Subsystem
  PS-Simulink Converter : nesl_utility/PS-Simulink Converter  PhysicalDomain=network_engine_domain  SubClassName=ps_output  LeftPortType=input  RightPortType=output  PseudoPeriodic=off  Frequencies=[]  Unit=inherit  AffineConversion=off
      settings: SourceProductBaseCode=PW,SS
  PS-Simulink Converter1 : nesl_utility/PS-Simulink Converter  PhysicalDomain=network_engine_domain  SubClassName=ps_output  LeftPortType=input  RightPortType=output  PseudoPeriodic=off  Frequencies=[]  Unit=inherit  AffineConversion=off
      settings: SourceProductBaseCode=PW,SS
  Sphere to Plane Force1 : Contact_Forces_Lib/3D/Sphere to Plane Force  sphere_rad=contact_point_radius  plane_lenx=plane_x  plane_leny=plane_y  plane_depth=height_plane/2  force_law=Linear  k_contact=contact_stiffness  b_contact=contact_damping  pen_full_damp_F=1e-4  pen_exponent=1  custom_param_1=1  custom_param_2=1  friction_law=Stick-Slip Continuous  mu_kinetic=mu_k  mu_static=mu_s  v_thr=mu_vth  vis_on=on  vis_opc_en=0  vis_len_plaBz=0.005  vis_clr=[0.9 0.2 0.2]  vis_opc=0.7
  Sphere to Plane Force2 : Contact_Forces_Lib/3D/Sphere to Plane Force  sphere_rad=contact_point_radius  plane_lenx=plane_x  plane_leny=plane_y  plane_depth=height_plane/2  force_law=Linear  k_contact=contact_stiffness  b_contact=contact_damping  pen_full_damp_F=1e-4  pen_exponent=1  custom_param_1=1  custom_param_2=1  friction_law=Stick-Slip Continuous  mu_kinetic=mu_k  mu_static=mu_s  v_thr=mu_vth  vis_on=off  vis_opc_en=0  vis_len_plaBz=0.005  vis_clr=[0.9 0.2 0.2]  vis_opc=0.7
  Sphere to Plane Force3 : Contact_Forces_Lib/3D/Sphere to Plane Force  sphere_rad=contact_point_radius  plane_lenx=plane_x  plane_leny=plane_y  plane_depth=height_plane/2  force_law=Linear  k_contact=contact_stiffness  b_contact=contact_damping  pen_full_damp_F=1e-4  pen_exponent=1  custom_param_1=1  custom_param_2=1  friction_law=Stick-Slip Continuous  mu_kinetic=mu_k  mu_static=mu_s  v_thr=mu_vth  vis_on=off  vis_opc_en=0  vis_len_plaBz=0.005  vis_clr=[0.9 0.2 0.2]  vis_opc=0.7
  Sphere to Plane Force4 : Contact_Forces_Lib/3D/Sphere to Plane Force  sphere_rad=contact_point_radius  plane_lenx=plane_x  plane_leny=plane_y  plane_depth=height_plane/2  force_law=Linear  k_contact=contact_stiffness  b_contact=contact_damping  pen_full_damp_F=1e-4  pen_exponent=1  custom_param_1=1  custom_param_2=1  friction_law=Stick-Slip Continuous  mu_kinetic=mu_k  mu_static=mu_s  v_thr=mu_vth  vis_on=off  vis_opc_en=0  vis_len_plaBz=0.005  vis_clr=[0.9 0.2 0.2]  vis_opc=0.7
  Subsystem : Subsystem
  To Workspace : ToWorkspace  VariableName=LFAnkle_measures  SaveFormat=Timeseries  SampleTime=-1
  To Workspace1 : ToWorkspace  VariableName=LFKnee_measures  SaveFormat=Timeseries  SampleTime=-1
  To Workspace2 : ToWorkspace  VariableName=LFHip_measures  SaveFormat=Timeseries  SampleTime=-1
  Upper Leg1 : sm_lib/Body Elements/Cylindrical Solid  GraphicAmbientColor=[0.15 0.15 0.15 1.0]  BasedOnType=Density  CenterOfMass=[0 0 0]  CenterOfMassUnits=m  GraphicDiffuseColor=[0.5 0.5 0.5]  CylinderLength=lower_leg_length  CylinderLengthUnits=cm  CylinderRadius=leg_radius  CylinderRadiusUnits=cm  Density=1000  DensityUnits=kg/m^3  DoExposeReferenceFrame=on  GraphicEmissiveColor=[0.0 0.0 0.0 1.0]  ExportEntireGeometry=off  SerializedFrames=<Frames/>  MarkerShape=Sphere  MarkerSize=10  GraphicType=FromGeometry  InertiaType=CalculateFromGeometry  Mass=1  MassUnits=kg  MomentsOfInertia=[1 1 1]  MomentsOfInertiaUnits=kg*m^2  GraphicOpacity=1.0  ProductsOfInertia=[1 1 1]  ProductsOfInertiaUnits=kg*m^2  GraphicShininess=75  GraphicSpecularColor=[0.5 0.5 0.5 1.0]  GraphicVisPropType=SimpleVisualProperties
  Upper leg to Hip1 : sm_lib/Frames and Transforms/Rigid Transform  TranslationMethod=Cartesian  TranslationStandardOffset=5  TranslationLengthUnit=cm  TranslationStandardAxis=+Z  TranslationCartesianOffset=[0 0 upper_leg_length/2]  TranslationROffset=0  TranslationROffsetUnits=m  TranslationZOffset=0  TranslationZOffsetUnits=m  TranslationThetaOffset=0  TranslationThetaOffsetUnits=deg  RotationMethod=StandardAxis  RotationAngleUnits=deg  RotationStandardAxis=+X  RotationAngle=90  RotationArbitraryAxis=[0 0 1]  FollAlignAxisA=+X  BaseAlignAxisA=+Y  FollAlignAxisB=+Y  BaseAlignAxisB=+Z  RotationSequenceAxes=FollowerAxes  RotationSequence=XYX  RotationSequenceAngles=[0 0 0]  RotationSequenceAnglesUnits=deg  RotationMatrix=[1 0 0; 0 1 0; 0 0 1]
  Upper leg LF : PMIOPort  Side=Left
  Lower leg LF : PMIOPort  Port=2  Side=Left
  Foot LF : PMIOPort  Port=3  Side=Left
  G : PMIOPort  Port=4  Side=Right
  H : PMIOPort  Port=5  Side=Right
  "Meas L " : Outport  VectorParamsAs1DForOutWhenUnconnected=off
  Outport : Outport  Port=2
  Outport1 : Outport  Port=3
  Outport2 : Outport  Port=4
  Outport4 : Outport  Port=5
  Outport5 : Outport  Port=6
  Outport3 : Outport  Port=7
  wires:
  Sphere to Plane Force4/1 -> "Contact Forces "/3(In3)
  Sphere to Plane Force2/1 -> "Contact Forces "/4(In4)
  Sphere to Plane Force3/1 -> "Contact Forces "/2(In2)
  Sphere to Plane Force1/1 -> "Contact Forces "/1(In1)
  "Contact Forces "/2(Out2) -> Measuring Component/3(Fr)
  "Contact Forces "/1(Out1) -> Measuring Component/1(Fn)
  Ankle and Motor/1(meas) -> To Workspace/1, Measuring Component/5(Ankle)
  Measuring Component/1(Meas) -> "Meas L "/1
  tddLF/1 -> MATLAB Function2/1(tddLF)
  Knee/1(meas) -> To Workspace1/1, Measuring Component/4(Knee)
  Hip/1(meas) -> Measuring Component/2(Hip), To Workspace2/1
  MATLAB Function2/3(tddLF_ankle) -> Ankle and Motor/1(tddLF_ankle)
  MATLAB Function2/2(tddLF_knee) -> Knee/1(tddLF_knee)
  MATLAB Function2/1(tddLF_hip) -> Hip/1(tddLF_hip)
  Ankle and Motor/2(Outport) -> Subsystem/1(qab)
  In2/1 -> Subsystem/2(Qquat)
  PS-Simulink Converter1/1 -> Subsystem/3(qkb)
  PS-Simulink Converter/1 -> Subsystem/4(qhb)
  Subsystem/1(Outport) -> Outport/1
  Knee/2(Outport) -> Subsystem/6(td2), MATLAB Function/2(knee)
  Hip/2(Outport) -> Subsystem/5(td1), MATLAB Function/3(hip)
  MATLAB Function/1(tdRF) -> Outport1/1
  vlinks/1 -> Subsystem/9(vlinks)
  v_torso/1 -> Subsystem/10(v_torso)
  w_torso/1 -> Subsystem/8(w_torso)
  Ankle and Motor/3(Outport1) -> Subsystem/7(td3), MATLAB Function/1(ankle)
  Subsystem/2(Outport1) -> Outport2/1
  Ankle and Motor/4(Outport2) -> MATLAB Function1/1(ankle)
  "Contact Forces "/4(Outport1) -> Outport5/1
  "Contact Forces "/3(Outport) -> Outport4/1
  theta_2d_des/1 -> MATLAB Function3/1(theta_2d_des)
  MATLAB Function3/1(t2ddhip) -> Hip/2(t2ddhip)
  MATLAB Function3/2(t2ddknee) -> Knee/2(t2ddknee)
  MATLAB Function3/3(t2ddankle) -> Ankle and Motor/2(t2ddankle)
  Knee/3(Outport1) -> MATLAB Function1/2(knee)
  Hip/3(Outport1) -> MATLAB Function1/3(hip)
  MATLAB Function1/1(t2dLF) -> Outport3/1
  Subsystem/3(Outport2) -> "Contact Forces "/5(Qd3g)
  connections:
  Lower Leg to Knee1/LConn1 -- Lower Leg1/RConn1 -- Lower leg LF/RConn1 -- Ankle to Lower Leg1/RConn1
  Ankle to Lower Leg1/LConn1 -- Ankle and Motor/RConn1
  Upper leg to Hip1/LConn1 -- Upper leg LF/RConn1 -- Upper Leg1/RConn1 -- Knee to Upper Leg1/RConn1
  Hip to World1/RConn1 -- H/RConn1
  Ankle and Motor/LConn1 -- Foot to Ankle1/RConn1
  Sphere to Plane Force3/LConn1 -- Foot1/LConn2
  Sphere to Plane Force1/LConn1 -- Foot1/LConn1
  Foot1/RConn2 -- Sphere to Plane Force4/LConn1
  Sphere to Plane Force4/RConn1 -- Sphere to Plane Force2/RConn1 -- G/RConn1 -- Sphere to Plane Force3/RConn1 -- Sphere to Plane Force1/RConn1
  Sphere to Plane Force2/LConn1 -- Foot1/RConn1
  Foot1/LConn3 -- Foot LF/RConn1 -- Foot to Ankle1/LConn1
  Knee to Upper Leg1/LConn1 -- Knee/RConn1
  Knee/LConn1 -- Lower Leg to Knee1/RConn1
  PS-Simulink Converter1/LConn1 -- Knee/LConn2
  Hip/LConn1 -- Upper leg to Hip1/RConn1
  Hip to World1/LConn1 -- Hip/RConn1
  PS-Simulink Converter/LConn1 -- Hip/LConn2
